simulink model "scratch_model"  (R2024b)
settings: Solver=VariableStepAuto  StartTime=0.0  StopTime=10.0  MaxStep=1e-4  RelTol=1e-3
libraries: eeGeneralControl x1
settings Model: Creator=baolo  LastModifiedBy=baolo

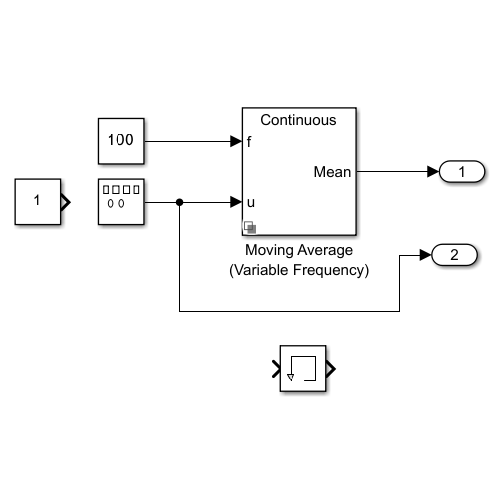
[thumbnail: Simulink's stored preview of the top-level diagram]
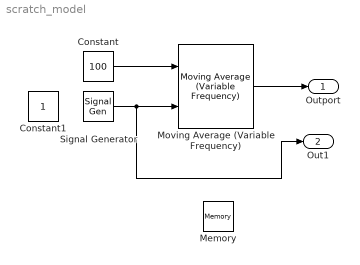
== system scratch_model ==
  Constant : Constant  Value=100
  Constant1 : Constant
  Memory : Memory
  Moving Average (Variable Frequency) : eeGeneralControl/Moving Average (Variable Frequency)  VariantControl=Variant1  LabelModeActiveChoice=Continuous  f0=60  fmin=30  x0=0  BufferSize=20000  Ts=0
      settings: LibrarySourceBlock=|
      | ee_sl_lib/General Control/Moving Average
      | (Variable Frequency)
  Signal Generator : SignalGenerator  Frequency=100
  Outport : Outport
  Out1 : Outport  Port=2
  wires:
  Constant/1 -> Moving Average (Variable Frequency)/1
  Signal Generator/1 -> Out1/1, Moving Average (Variable Frequency)/2
  Moving Average (Variable Frequency)/1 -> Outport/1
